simulink model "DCMOTORDISK"  (R2018b)
settings: Solver=ode15s  StartTime=0.0  StopTime=120  RelTol=1e-3  AbsTol=1e-3  EnableMultiTasking=on
libraries: fl_lib x6, nesl_utility x5, simulink x1, SignalEditorBlockLib x1, elec_lib x1
CloseFcn:
  | try,close(h1_elec_motor_dc_pwm),end
  | clear h1_elec_motor_dc_pwm
  | 
  | clear simlog_elec_motor_dc_pwm
  | clear logsout_elec_motor_dc_pwm
Description:
  | PWM-Controlled DC Motor
  | 
  | Copyright 2008-2018 The MathWorks, Inc.
settings Model: Creator=MathWorks  LastModifiedBy=pirana
settings SolverCC: AutoScaleAbsTol=off
settings DataIOCC: LimitDataPoints=on  MaxDataPoints=10000  SaveFormat=Array  SignalLoggingSaveFormat=ModelDataLogs  SignalLoggingName=logsout_elec_motor_dc_pwm
settings OptimizationCC: ExpressionDepthLimit=2147483647  InitFltsAndDblsToZero=on  LifeSpan=inf
settings DebuggingCC: UnderspecifiedInitializationDetection=Classic  MergeDetectMultiDrivingBlocksExec=none  FcnCallInpInsideContextMsg=warning  StateNameClashWarn=warning  LibraryContextMissingDiagnostic=none  SFUnexpectedBacktrackingDiag=warning  SFNoUnconditionalDefaultTransitionDiag=warning  SFExecutionAtInitializationDiag=none
settings HardwareCC: ProdBitPerPointer=32  ProdBitPerSizeT=32  ProdBitPerPtrDiffT=32  ProdLargestAtomicFloat=None  ProdIntDivRoundTo=Undefined  ProdEndianess=Unspecified  ProdWordSize=32  ProdHWDeviceType=32-bit Generic
settings ModelReferenceCC: PropagateSignalLabelsOutOfModel=off
settings SFSimCC: SimUseLocalCustomCode=off
settings RTWCC: RTWUseLocalCustomCode=off
settings CodeAppCC: StateflowObjectComments=on
settings GRTTargetCC: TargetLangStandard=C89/C90 (ANSI)  GeneratePreprocessorConditionals=Disable all  CombineOutputUpdateFcns=off  GRTInterface=on
settings ConfigComp: CovMetricSettings=dw  CovHtmlReporting=on  CovSaveCumulativeToWorkspaceVar=on  CovSaveSingleToWorkspaceVar=on  CovExternalEMLEnable=off  CovSFcnEnable=off
settings SimscapeCC: SimscapeLogType=all  SimscapeLogSimulationStatistics=on  SimscapeLogName=simlog_elec_motor_dc_pwm  SimscapeLogDataHistory=10000

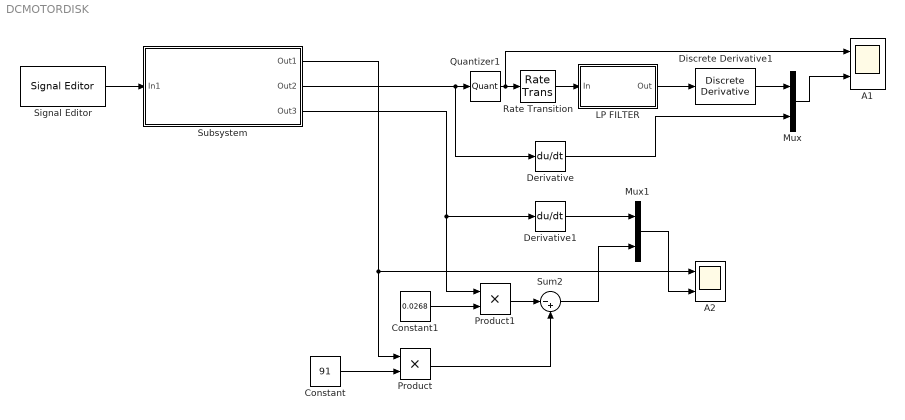
== system DCMOTORDISK ==
  A1 : Scope  NumInputPorts=2
  A2 : Scope  NumInputPorts=2
  Constant : Constant  Value=91
  Constant1 : Constant  Value=0.0268
  Derivative : Derivative
  Derivative1 : Derivative
  Discrete Derivative1 : simulink/Discrete/Discrete Derivative  gainval=1.0  ICPrevScaledInput=0.0  OutMin=[]  OutMax=[]  OutDataType=fixdt(1, 16)  OutScaling=2^-10  DoSatur=off
  LP FILTER : Subsystem  Tag=BlockMethodSubSystem
  Mux : Mux  Inputs=2
  Mux1 : Mux  Inputs=2
  Product : Product
  Product1 : Product
  Quantizer1 : Quantizer  QuantizationInterval=0.0061
  Rate Transition : RateTransition  OutPortSampleTime=0.0001
  Signal Editor : SignalEditorBlockLib/Signal Editor  FileName=Signal.mat  ActiveScenario=Scenario  ActiveSignal=Signal  IsBus=off  OutputBusObjectStr=Bus: BusObject  SampleTime=0  Interpolate=off  ZeroCross=off  OutputAfterFinalValue=Setting to zero  Unit=inherit
  Subsystem : Subsystem
  Sum2 : Sum  Inputs=|-+
  wires:
  Signal Editor/1 -> Subsystem/1(In1)
  Subsystem/1(Out1) -> Product/1, A2/1
  Subsystem/2(Out2) -> Derivative/1, Quantizer1/1
  Derivative/1 -> Mux/2
  Mux/1 -> A1/2
  Subsystem/3(Out3) -> Product1/1, Derivative1/1
  Product/1 -> Sum2/2
  Constant1/1 -> Product1/2
  Constant/1 -> Product/2
  Product1/1 -> Sum2/1
  Sum2/1 -> Mux1/2
  Mux1/1 -> A2/2
  Derivative1/1 -> Mux1/1
  Rate Transition/1 -> LP FILTER/1(In)
  LP FILTER/1(Out) -> Discrete Derivative1/1
  Discrete Derivative1/1 -> Mux/1
  Quantizer1/1 -> A1/1, Rate Transition/1

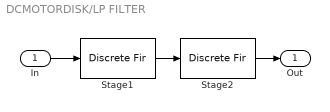
== system DCMOTORDISK/LP FILTER ==
  In : Inport
  Stage1 : DiscreteFir  Tag=BlockMethodSubSystem  Coefficients=[-0.00199176357174310351 -0.00530450815012495358 -0.00950904683591792532 -0.0118117877261882422 -0.00798237885539230044 0.00626240257079945309 0.0330636315806409897 0.0704895675201800964 0.112018428473465742 0.14803803569995988 0.169011346165353848 0.169011346165353848 0.14803803569995988 0.112018428473465742 0.0704895675201800964 0.0330636315806409897 0.00626240257079945309 -0.00798237885539230044 -0.0118117877261882422 -0.00950904683591792532 -0.00530450815012495358 -0.00199176357174310351]  InputProcessing=Columns as channels (frame based)
  Stage2 : DiscreteFir  Tag=BlockMethodSubSystem  Coefficients=[0.000211638813508944449 0 0 0 0 -0.00191887158392450331 0 0 0 0 -0.00480866362502560454 0 0 0 0 -0.00567328345390206989 0 0 0 0 -0.000542412375559235549 0 0 0 0 0.0101759749332177817 0 0 0 0 0.0183947823331915665 0 0 0 0 0.012300284360340915 0 0 0 0 -0.0123410580554456292 0 0 0 0 -0.0419986004222386786 0 0 0 0 -0.0477281139772199603 0 0 0 0 -0.00331824393029788584 0 0 0 0 0.0917895196921782175 0 0 0 0 0.203541416989306861 0 0 0 0 0.279096039103617244 0 0 0 0 0.279096039103617244 0 0 0 0 0.203541416989306861 0 0 0 0 0.0917895196921782175 0 0 0 0 -0.00331824393029788584 0 0 0 0 -0.0477281139772199603 0 0 0 0 -0.0419986004222386786 0 0 0 0 -0.0123410580554456292 0 0 0 0 0.012300284360340915 0 0 0 0 0.0183947823331915665 0 0 0 0 0.0101759749332177817 0 0 0 0 -0.000542412375559235549 0 0 0 0 -0.00567328345390206989 0 0 0 0 -0.00480866362502560454 0 0 0 0 -0.00191887158392450331 0 0 0 0 0.000211638813508944449]  InputProcessing=Columns as channels (frame based)
  Out : Outport
  wires:
  In/1 -> Stage1/1
  Stage1/1 -> Stage2/1
  Stage2/1 -> Out/1

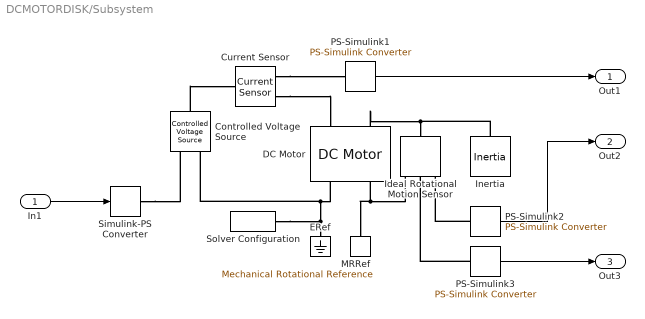
== system DCMOTORDISK/Subsystem ==
  In1 : Inport
  Controlled Voltage Source : fl_lib/Electrical/Electrical Sources/Controlled Voltage Source
  Current Sensor : fl_lib/Electrical/Electrical Sensors/Current Sensor
      settings: SourceProductName=Foundation Library
  DC Motor : elec_lib/Actuators & Drivers/Rotational Actuators/DC Motor  parameterization=2  Ra=3.38 Ohm  La=0.01 H  emf_or_torque=1  Kv=0.029 V/(rad/s)  Ki=6.876e-04 N*m/A  T_stall=0.02 N*m  w_max=6000 rpm  w_rated=3000 rpm  P_rated=10 W  V_rated=12 V  J=0.00001 kg*m^2  lam_param=2  lam=0.5e-5 N*m/(rad/s)  i_noload=180 mA  V_i_noload=12 V  speed0=0 rad/s  alpha=0.00393 1/K  Tmeas=25 degC  thermal_mass=100 J/K  initial_temperature=25 degC
  ERef : fl_lib/Electrical/Electrical Elements/Electrical Reference
      settings: SourceProductName=Foundation Library
  Ideal Rotational Motion Sensor : fl_lib/Mechanical/Mechanical Sensors/Ideal Rotational Motion Sensor  offset=0 deg
      settings: SourceProductName=Foundation Library
  Inertia : fl_lib/Mechanical/Rotational Elements/Inertia  inertia=0.00016923972 kg*m^2  w_specify=off  w_priority=High  w=0 rad/s  w_nominal_specify=off  w_nominal_unit=rad/s  w_nominal_value=1  t_specify=off  t_priority=None  t=0 N*m  t_nominal_specify=off  t_nominal_unit=N*m  t_nominal_value=1
  MRRef : fl_lib/Mechanical/Rotational Elements/Mechanical Rotational Reference
      settings: SourceProductName=Foundation Library
  PS-Simulink1 : nesl_utility/PS-Simulink Converter  PhysicalDomain=network_engine_domain  SubClassName=ps_output  LeftPortType=input  RightPortType=output  PseudoPeriodic=off  Frequencies=[]  Unit=A  AffineConversion=off
  PS-Simulink2 : nesl_utility/PS-Simulink Converter  PhysicalDomain=network_engine_domain  SubClassName=ps_output  LeftPortType=input  RightPortType=output  PseudoPeriodic=off  Frequencies=[]  Unit=rad  AffineConversion=off
  PS-Simulink3 : nesl_utility/PS-Simulink Converter  PhysicalDomain=network_engine_domain  SubClassName=ps_output  LeftPortType=input  RightPortType=output  PseudoPeriodic=off  Frequencies=[]  Unit=rad/s  AffineConversion=off
  Simulink-PS Converter : nesl_utility/Simulink-PS Converter  PhysicalDomain=network_engine_domain  SubClassName=ps_input  LeftPortType=input  RightPortType=output  PseudoPeriodic=off  Frequencies=[]  NoiseDistribution=none  NoiseParameters=[]  Unit=1  AffineConversion=off  FilteringAndDerivatives=provide  SimscapeFilterOrder=1  InputFilterTimeConstant=0.001  UdotUserProvided=0
  Solver Configuration : nesl_utility/Solver Configuration  PhysicalDomain=network_engine_domain  SubClassName=solver  LeftPortType=input  RightPortType=generic  Tones=[]  Harmonics=[]  SimulateNoise=off  Profile=off  UseLocalSampling=off  EnableSwitchedLinearOptims=on  FrequencyDomain=off  UseCCode=off  RelTol=0.001  AbsTol=1e-06  MinStep=1e-09  ToWorkspace=off  RevertToSquareIcSolve=off  NumHomotopyIterations=100  PhasorMode=off  PhasorModeNumHarmonics=1  DoDC=off  ResidualTolerance=1e-9  UseLocalSolver=off  LocalSolverChoice=NE_BACKWARD_EULER_ADVANCER  LocalSolverSampleTime=.001  DoFixedCost=off  MaxNonlinIter=3  MaxModeIter=2  LinearAlgebra=Sparse  EquationFormulation=NE_TIME_EF  DelaysMemoryBudget=1024  AutomaticFiltering=on  FilteringTimeConstant=0.001  PartitionStorageMethod=AS_NEEDED  PartitionMemoryBudget=1024
  Out1 : Outport
  Out2 : Outport  Port=2
  Out3 : Outport  Port=3
  wires:
  In1/1 -> Simulink-PS Converter/1
  PS-Simulink2/1 -> Out2/1
  PS-Simulink1/1 -> Out1/1
  PS-Simulink3/1 -> Out3/1
  connections:
  Current Sensor/RConn1 -- PS-Simulink1/LConn1
  Controlled Voltage Source/RConn2 -- DC Motor/RConn1 -- Solver Configuration/RConn1 -- ERef/LConn1
  PS-Simulink2/LConn1 -- Ideal Rotational Motion Sensor/RConn3
  Current Sensor/RConn2 -- DC Motor/LConn1
  DC Motor/LConn2 -- Inertia/LConn1 -- Ideal Rotational Motion Sensor/LConn1
  DC Motor/RConn2 -- MRRef/LConn1 -- Ideal Rotational Motion Sensor/RConn1
  Simulink-PS Converter/RConn1 -- Controlled Voltage Source/RConn1
  Controlled Voltage Source/LConn1 -- Current Sensor/LConn1
  PS-Simulink3/LConn1 -- Ideal Rotational Motion Sensor/RConn2
